simulink model "miniproject"  (R2021a)
settings: Solver=VariableStepAuto  StartTime=0.0  StopTime=0.5  RelTol=1e-3
libraries: spsIGBTDiodeLib x6, simulink x3, spsDCVoltageSourceLib x1, simrfV2_lib x1, spsSawtoothGeneratorLib x1, spsThreePhaseVIMeasurementLib x1, spsThreePhaseParallelRLCBranchLib x1, spspowerguiLib x1
settings Model: Creator=mluser  LastModifiedBy=mluser

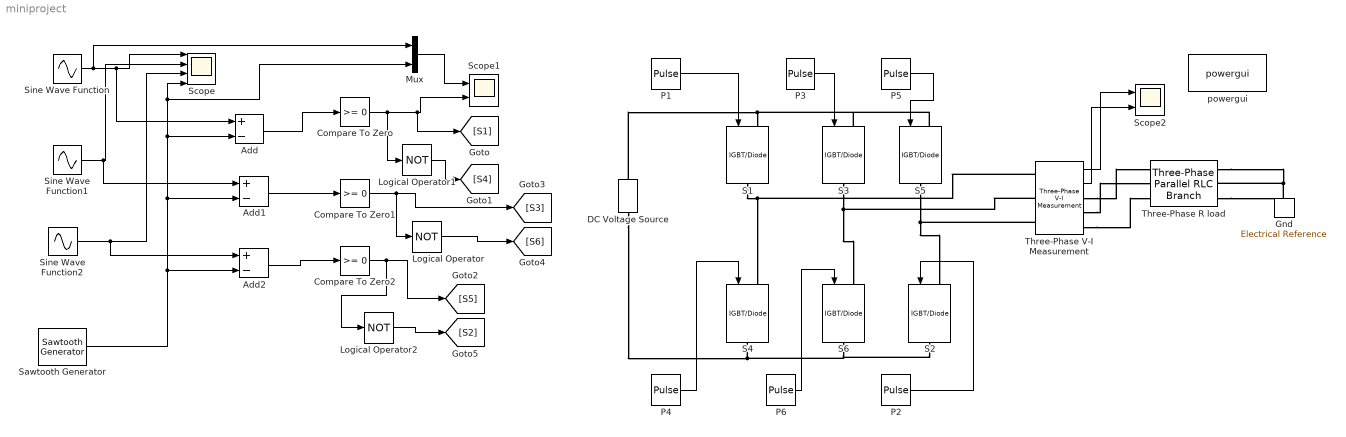
== system miniproject ==
  Add : Sum  Inputs=+-
  Add1 : Sum  Inputs=+-
  Add2 : Sum  Inputs=+-
  Compare To Zero : simulink/Logic and Bit Operations/Compare To Zero  relop=>=  OutDataTypeStr=boolean
  Compare To Zero1 : simulink/Logic and Bit Operations/Compare To Zero  relop=>=  OutDataTypeStr=boolean
  Compare To Zero2 : simulink/Logic and Bit Operations/Compare To Zero  relop=>=  OutDataTypeStr=boolean
  DC Voltage Source : spsDCVoltageSourceLib/DC Voltage Source  Amplitude=230  Measurements=None
  Gnd : simrfV2_lib/Elements/Electrical Reference
      settings: SourceProductBaseCode=RB  InternalSimscapePortConfiguration="{\"Bottom\":[],\"Left\":[{\"id\":\"V\",\"label\":\"\",\"type\":\"foundation.rf.circuitenvelope\"}],\"Right\":[],\"Top\":[]}"
  Logical Operator : Logic  Operator=NOT  AllPortsSameDT=off  OutDataTypeStr=boolean
  Logical Operator1 : Logic  Operator=NOT  AllPortsSameDT=off  OutDataTypeStr=boolean
  Logical Operator2 : Logic  Operator=NOT  AllPortsSameDT=off  OutDataTypeStr=boolean
  Mux : Mux  Inputs=2
  P1 : DiscretePulseGenerator  PulseType=Time based  Period=0.02  PulseWidth=50
  P2 : DiscretePulseGenerator  PulseType=Time based  Period=0.02  PulseWidth=50  PhaseDelay=60*0.02/360
  P3 : DiscretePulseGenerator  PulseType=Time based  Period=0.02  PulseWidth=50  PhaseDelay=120*0.02/360
  P4 : DiscretePulseGenerator  PulseType=Time based  Period=0.02  PulseWidth=50  PhaseDelay=180*0.02/360
  P5 : DiscretePulseGenerator  PulseType=Time based  Period=0.02  PulseWidth=50  PhaseDelay=240*0.02/360
  P6 : DiscretePulseGenerator  PulseType=Time based  Period=0.02  PulseWidth=50  PhaseDelay=300*0.02/360
  S{1..6} (6 alike) : spsIGBTDiodeLib/IGBT//Diode  Ron=1e-3  Rs=1e5  Cs=inf  Measurements=off
  Sawtooth Generator : spsSawtoothGeneratorLib/Sawtooth Generator  Freq=1e3  Phase=180  Ts=0
  Scope : Scope  NumInputPorts=4
  Scope1 : Scope  NumInputPorts=2
  Scope2 : Scope  NumInputPorts=2
  Sine Wave Function : Sin  TimeSource=Use external signal  Frequency=2*pi*50  SampleTime=0
  Sine Wave Function1 : Sin  TimeSource=Use external signal  Frequency=2*pi*50  Phase=2*pi/3  SampleTime=0
  Sine Wave Function2 : Sin  TimeSource=Use external signal  Frequency=2*pi*50  Phase=4*pi/3  SampleTime=0
  Three-Phase V-I Measurement : spsThreePhaseVIMeasurementLib/Three-Phase V-I Measurement  VoltageMeasurement=phase-to-phase  SetLabelV=off  LabelV=Vabc  Vpu=off  VpuLL=off  CurrentMeasurement=yes  SetLabelI=off  LabelI=Iabc  Ipu=off  Pbase=100e6  Vbase=500e3  OutputType=Complex  PhasorSimulation=off  PSBequivalent=0
  Three-Phase R load : spsThreePhaseParallelRLCBranchLib/Three-Phase Parallel RLC Branch  LConnTagsString=A|B|C  RConnTagsString=A|B|C  BranchType=R  Resistance=1  Inductance=1e-3  Capacitance=1e-6  Measurements=None
      settings: SourceProductBaseCode=PS
  powergui : spspowerguiLib/powergui  Priority=1  SimulationMode=Discrete  SampleTime=50e-6  frequency=60  Iterations=50  frequencyindice=0  Pbase=100e6  ErrMax=1e-4  UnitsV=kV  UnitsW=MW  buscounter=0  FunctionMessages=off  echomessages=off  EnableUseOfTLC=off  CurrentSourceSwitches=off  DisableSnubberDevices=off  DisableRonSwitches=off  DisableVfSwitches=off  DisplayEquations=off  AutomaticDiscreteSolvers=off  SolverType=Tustin/Backward Euler (TBE)  Interpol=off  ExternalGateDelay=off  methode=off  Ts=100  x0status=blocks  SPID=on  SwTol=0  HookPort=off  NonlinearTolerance=1e-4  nMaxIteration=100  ContinueOnMaxIteration=off  RestoreLinks=warning  ResistiveCurrentMeasurement=off  Frange=[0:2:500]  Ylog=off  Xlog=on  ShowGrid=off  save=off  variable=ZData  structure=0  ZoomFFT=off  StartTime=0.0  cycles=1  DisplayStyle=1  fundamental=60  FreqAxis=off  MaxFrequency=1000  frequencyindicesteady=1  RmsSteady=1  display=off
  wires:
  Sine Wave Function/1 -> Mux/1, Add/1, Scope/1
  Sine Wave Function1/1 -> Add1/1, Scope/2
  Sine Wave Function2/1 -> Add2/1, Scope/3
  Sawtooth Generator/1 -> Add2/2, Add1/2, Add/2, Mux/2, Scope/4
  Add/1 -> Compare To Zero/1
  Add1/1 -> Compare To Zero1/1
  Add2/1 -> Compare To Zero2/1
  Mux/1 -> Scope1/1
  Compare To Zero/1 -> Logical Operator1/1, [S1], Scope1/2
  Compare To Zero1/1 -> Logical Operator/1, [S3]
  Compare To Zero2/1 -> Logical Operator2/1, [S5]
  Logical Operator1/1 -> [S4]
  Logical Operator/1 -> [S6]
  Logical Operator2/1 -> [S2]
  P1/1 -> S1/1
  P2/1 -> S2/1
  P3/1 -> S3/1
  P4/1 -> S4/1
  P5/1 -> S5/1
  P6/1 -> S6/1
  Three-Phase V-I Measurement/1 -> Scope2/1
  Three-Phase V-I Measurement/2 -> Scope2/2
  connections:
  S1/RConn1 -- Three-Phase V-I Measurement/LConn1 -- S4/LConn1
  DC Voltage Source/RConn1 -- S5/LConn1 -- S3/LConn1 -- S1/LConn1
  Three-Phase V-I Measurement/RConn1 -- Three-Phase R load/LConn1
  Three-Phase V-I Measurement/RConn2 -- Three-Phase R load/LConn2
  Three-Phase V-I Measurement/RConn3 -- Three-Phase R load/LConn3
  Three-Phase R load/RConn1 -- Three-Phase R load/RConn3 -- Three-Phase R load/RConn2
  DC Voltage Source/LConn1 -- S2/RConn1 -- S6/RConn1 -- S4/RConn1
  S3/RConn1 -- Three-Phase V-I Measurement/LConn2 -- S6/LConn1
  S5/RConn1 -- Three-Phase V-I Measurement/LConn3 -- S2/LConn1
